simulink model "usv_model"  (R2016a)
settings: Solver=VariableStepAuto  StartTime=0.0  StopTime=10  RelTol=1e-3
libraries: simulink x1
settings Model: Creator=ASUS  LastModifiedBy=ASUS

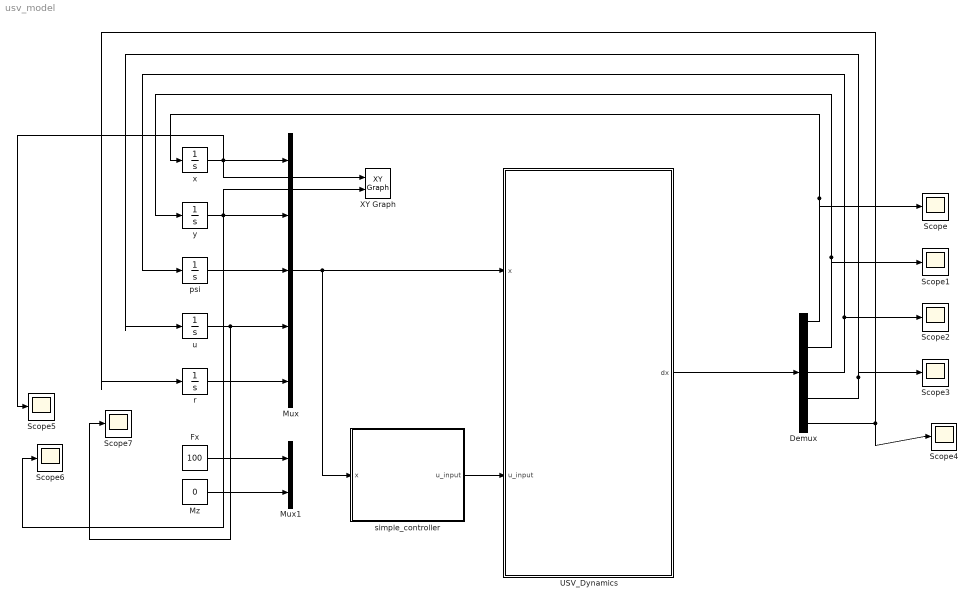
== system usv_model ==
  Demux : Demux  Outputs=5
  "Fx " : Constant  Value=100
  Mux : Mux  Inputs=5
  Mux1 : Mux  Inputs=2
  Mz : Constant  Value=0
  Scope{,1..7} (8 alike) : Scope
  "USV_Dynamics " : MATLAB Function  TreatAsAtomicUnit=on
  XY Graph : simulink/Sinks/XY Graph  xmin=-100  xmax=100  ymin=-100  ymax=100  st=-1
  psi : Integrator
  r : Integrator
  simple_controller : MATLAB Function  TreatAsAtomicUnit=on
  u : Integrator
  x : Integrator
  y : Integrator
  wires:
  y/1 -> Scope6/1, Mux/2, XY Graph/2
  psi/1 -> Mux/3
  u/1 -> Scope7/1, Mux/4
  r/1 -> Mux/5
  Mux/1 -> "USV_Dynamics "/1(x), simple_controller/1(x)
  "Fx "/1 -> Mux1/1
  Mz/1 -> Mux1/2
  Demux/4 -> Scope3/1, u/1
  "USV_Dynamics "/1(dx) -> Demux/1
  Demux/1 -> Scope/1, x/1
  Demux/2 -> Scope1/1, y/1
  Demux/3 -> Scope2/1, psi/1
  Demux/5 -> r/1, Scope4/1
  simple_controller/1(u_input) -> "USV_Dynamics "/2(u_input)
  x/1 -> Scope5/1, XY Graph/1, Mux/1

== matlab function usv_model/simple_controller ==
  data: x input size=[5 1]; u_input output size=[2 1]
function u_input = simple_controller(x)
    x_target = 100;
    y_target = 50;

    % Kontrol kazançları
    Kp = 100;
    Kd = 20;
    Kp_yaw = 500;
    Kd_yaw = 100;

    x_pos = x(1);
    y_pos = x(2);
    psi   = x(3);
    u     = x(4);
    r     = x(5);

    dx = x_target - x_pos;
    dy = y_target - y_pos;

    x_error = abs(dx);
    y_error = abs(dy);

    tolerance = 0.5;

    if x_error < tolerance && y_error < tolerance
        Fx = 0;
        Mz = 0;
    else
        yaw_target = atan2(dy, dx);
        yaw_error = mod(yaw_target - psi + pi, 2*pi) - pi;

        dist = sqrt(dx^2 + dy^2);

        max_yaw_error_for_forward = pi/6; % 30 derece

        if abs(yaw_error) > max_yaw_error_for_forward
            Fx = 0; % Önce dön
        else
            Fx = Kp * dist - Kd * u;
            Fx = max(Fx, 0);
        end

        Mz = Kp_yaw * yaw_error - Kd_yaw * r;
        Mz = min(max(Mz, -200), 200);
    end

    u_input = [Fx; Mz];
end

== matlab function usv_model/USV_Dynamics  ==
  data: x input size=[5 1]; dx output size=[5 1]; u_input input size=[2 1]
function dx = USV_Dynamics(x, u_input)
    % Basit 2D USV dinamiği
    % x = [X; Y; psi; u; r]
    % u_input = [Fx; Mz]
    
    % Araç parametreleri
    m = 50;      % kg
    Iz = 200;    % kg*m^2 - Atalet Momenti
    X_damp = 150;  % lineer sönüm - Eğer hala hız yüksek kalıyorsa X_damp değerini artırabilirsin.
    N_damp = 500; % yaw sönüm - Dönmede problem varsa N_damp değerini artır.

    % Girişler
    Fx = u_input(1); 
    Mz = u_input(2);
    
    % Durumlar
    psi = x(3); 
    u   = x(4); 
    r   = x(5);

    % Durum türevleri
    dx = zeros(5,1);
    dx(1) = u*cos(psi);       % X_dot
    dx(2) = u*sin(psi);       % Y_dot
    dx(3) = r;                % psi_dot
    dx(4) = (1/m)*(Fx - X_damp*u);     % u_dot
    dx(5) = (1/Iz)*(Mz - N_damp*r);    % r_dot
end
